simulink model "simulink_model"  (R2021a)
settings: Solver=VariableStepAuto  StartTime=0.0  StopTime=710  RelTol=1e-3
values from neighbouring files (symbols this model uses):
  C = S/rho/g    [model_parameters.m]
  g = 9.81    [model_parameters.m]
  G = (L1+h1-h3)*rho*g*I/p*1.08    (= 222.05302768)    [model_parameters.m]
  I = 1/Pmax/tau    (= 0.00378787878788)    [model_parameters.m]
  initial_condition = [initial_volumes ; 0]    [model_parameters.m]
  L1 = (1900+100 - 50 - 229)*1e-3    (= 1.721)    [model_parameters.m]
  rho = 998    [model_parameters.m]
  Rp = I / tau    (= 0.00789141414141)    [model_parameters.m]
  RT1 = pipe_resistance(L1, pipe_radius)*9    [model_parameters.m]
  RT2 = pipe_resistance(L2, pipe_radius) *2*2    [model_parameters.m]
  RT3 = pipe_resistance(L3, pipe_radius) *5    [model_parameters.m]
  S = [S1 S2 S3]    [model_parameters.m]
  Uset_max = sqrt(Pmax * Rp)    [model_parameters.m]
libraries: simulink x3
settings Model: Creator=vomi  LastModifiedBy=vomi

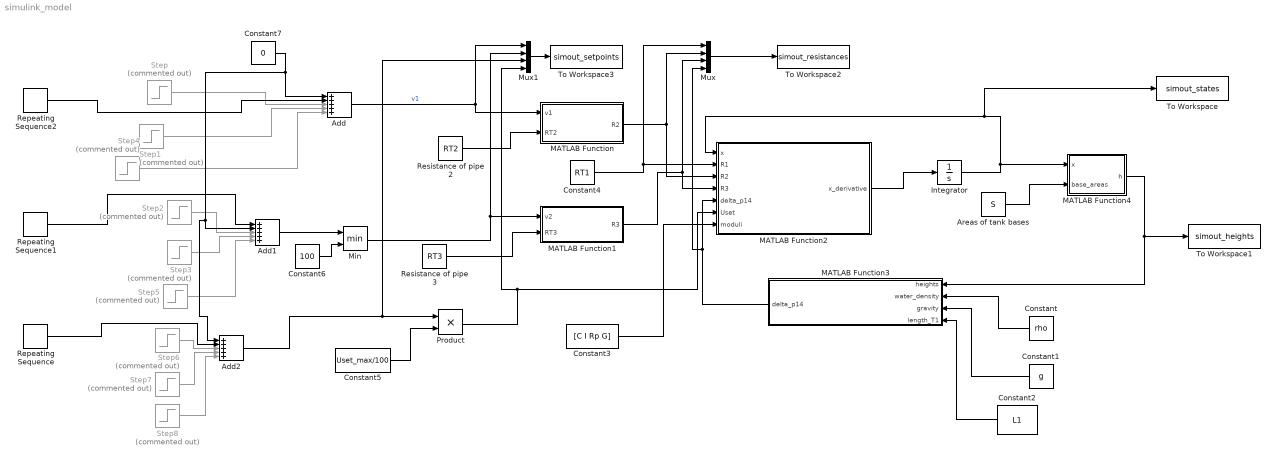
== system simulink_model ==
  Add : Sum  Inputs=+++++
  Add1 : Sum  Inputs=+++++
  Add2 : Sum  Inputs=+++++
  Areas of tank bases : Constant  Value=S
  Constant : Constant  Value=rho
  Constant1 : Constant  Value=g
  Constant2 : Constant  Value=L1
  Constant3 : Constant  Value=[C I Rp G]
  Constant4 : Constant  Value=RT1
  Constant5 : Constant  Value=Uset_max/100
  Constant6 : Constant  Value=100
  Constant7 : Constant  Value=0
  Integrator : Integrator  InitialCondition=initial_condition
  MATLAB Function : MATLAB Function  TreatAsAtomicUnit=on
  MATLAB Function1 : MATLAB Function  TreatAsAtomicUnit=on
  MATLAB Function2 : MATLAB Function  TreatAsAtomicUnit=on
  MATLAB Function3 : MATLAB Function  TreatAsAtomicUnit=on
  MATLAB Function4 : MATLAB Function  TreatAsAtomicUnit=on
  Min : MinMax  Inputs=2
  Mux : Mux
  Mux1 : Mux
  Product : Product
  Repeating Sequence : simulink/Sources/Repeating Sequence  rep_seq_t=event_times  rep_seq_y=pump_setpoints
  Repeating Sequence1 : simulink/Sources/Repeating Sequence  rep_seq_t=event_times  rep_seq_y=v2_setpoints
  Repeating Sequence2 : simulink/Sources/Repeating Sequence  rep_seq_t=event_times  rep_seq_y=v1_setpoints
  Resistance of pipe 2 : Constant  Value=RT2
  Resistance of pipe 3 : Constant  Value=RT3
  Step : Step  Commented=on  Time=50  SampleTime=0
  Step1 : Step  Commented=on  Time=100  After=-1  SampleTime=0
  Step2 : Step  Commented=on  Time=80  Before=15  After=80  SampleTime=0
  Step3 : Step  Commented=on  Time=120  After=-55  SampleTime=0
  Step4 : Step  Commented=on  Time=160  SampleTime=0
  Step5 : Step  Commented=on  Time=300  After=100  SampleTime=0
  Step6 : Step  Commented=on  Time=260  After=50  SampleTime=0
  Step7 : Step  Commented=on  Time=350  After=-20  SampleTime=0
  Step8 : Step  Commented=on  Time=400  After=-30  SampleTime=0
  To Workspace : ToWorkspace  VariableName=simout_states  SaveFormat=Structure With Time  SampleTime=-1
  To Workspace1 : ToWorkspace  VariableName=simout_heights  SaveFormat=Structure With Time  SampleTime=-1
  To Workspace2 : ToWorkspace  VariableName=simout_resistances  SaveFormat=Structure With Time  SampleTime=-1
  To Workspace3 : ToWorkspace  VariableName=simout_setpoints  SaveFormat=Structure With Time  SampleTime=-1
  wires:
  Add/1 -> Mux1/1, MATLAB Function/1(v1)  "v1"
  Step2/1 -> Add1/3
  MATLAB Function2/1(x_derivative) -> Integrator/1
  Integrator/1 -> MATLAB Function4/1(x), To Workspace/1, MATLAB Function2/1(x)
  MATLAB Function/1(R2) -> Mux/2, MATLAB Function2/3(R2)
  MATLAB Function1/1(R3) -> Mux/3, MATLAB Function2/4(R3)
  Add2/1 -> Mux1/3, Product/1
  MATLAB Function3/1(delta_p14) -> Mux/4, MATLAB Function2/5(delta_p14)
  MATLAB Function4/1(h) -> MATLAB Function3/1(heights), To Workspace1/1
  Resistance of pipe 2/1 -> MATLAB Function/2(RT2)
  Resistance of pipe 3/1 -> MATLAB Function1/2(RT3)
  Areas of tank bases/1 -> MATLAB Function4/2(base_areas)
  Constant/1 -> MATLAB Function3/2(water_density)
  Constant1/1 -> MATLAB Function3/3(gravity)
  Constant2/1 -> MATLAB Function3/4(length_T1)
  Constant3/1 -> MATLAB Function2/7(moduli)
  Constant4/1 -> Mux/1, MATLAB Function2/2(R1)
  Mux/1 -> To Workspace2/1
  Mux1/1 -> To Workspace3/1
  Step/1 -> Add/3
  Step1/1 -> Add/4
  Min/1 -> Mux1/2, MATLAB Function1/1(v2)
  Step3/1 -> Add1/4
  Step4/1 -> Add/5
  Step5/1 -> Add1/5
  Add1/1 -> Min/1
  Constant6/1 -> Min/2
  Constant7/1 -> Add1/2, Add2/1, Add/1
  Constant5/1 -> Product/2
  Product/1 -> MATLAB Function2/6(Uset), Mux1/4
  Step6/1 -> Add2/3
  Step7/1 -> Add2/4
  Step8/1 -> Add2/5
  Repeating Sequence/1 -> Add2/2
  Repeating Sequence1/1 -> Add1/1
  Repeating Sequence2/1 -> Add/2

== matlab function simulink_model/MATLAB Function1 ==
  data: v2 input; R3 output; RT3 input
function R3 = calculate_R3(v2, RT3)

R3 = RT3 * (100-20)/(max(v2, 20)-20);

== matlab function simulink_model/MATLAB Function ==
  data: v1 input; R2 output; RT2 input
function R2 = calculate_R2(v1, RT2)
    R2 = RT2/v1;
end

== matlab function simulink_model/MATLAB Function2 ==
  data: x input; R1 input; R2 input; R3 input; delta_p14 input; x_derivative output; Uset input; moduli input
function x_derivative = state_model(x, R1, R2, R3, delta_p14,Uset, moduli)

C1 = moduli(1);
C2 = moduli(2);
C3 = moduli(3);
I  = moduli(4);
Rp = moduli(5);
G  = moduli(6);


to_q1 = [-1/C1*(1/R1+1/R2), 1/C2/R2, 1/C3/R1, G/I/R1];
to_q2 = [1/C1/R2           , -1/C2*(1/R2+1/R3), 0 , 0];
to_q3 = [1/C1/R1, 1/C2/R3, -1/C3/R1, -G/I/R1];
%to_p = [G/C1/R1, 0, -G/C3/R1, -1/I*(Rp + G^2/R1)]; % Tekoucí voda ovlivňuje pumpu
to_p = [0, 0, 0, -Rp/I];

A = [to_q1; to_q2; to_q3; to_p];

% const_offset = [-1;0;1;G] * delta_p14 / R1; Tekoucí voda ovlivňuje pumpu
const_offset = [-1;0;1;0] * delta_p14 / R1;

setpoints = [0;0;0; Uset];

x_derivative = A * x + const_offset + setpoints;

== matlab function simulink_model/MATLAB Function3 ==
  data: heights input; delta_p14 output; water_density input; gravity input; length_T1 input
function delta_p14 = calculate_delta_p14(heights, water_density, gravity, length_T1)

rho = water_density;
g = gravity;

if heights(1) > 1e-4
    delta_p14 = rho*g*length_T1;
else
    delta_p14 = 0;
end

== matlab function simulink_model/MATLAB Function4 ==
  data: x input; h output; base_areas input
function h = volumes_to_heights(x, base_areas)

h = x(1:3)./base_areas;
